simulink model "C1"  (Simulink 7.4)
settings: Solver=ode45  StartTime=0.0  StopTime=30  MaxStep=0.1  AbsTol=1e-14
settings Model: Creator=Administrator  LastModifiedBy=Administrator

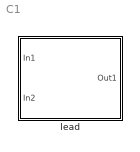
== system C1 ==
  lead : Subsystem

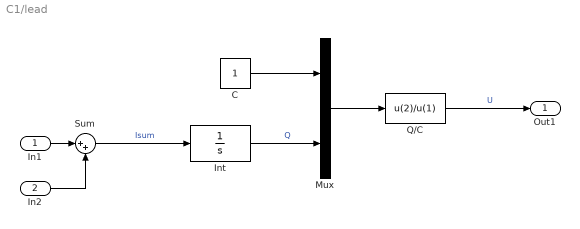
== system C1/lead ==
  In1 : Inport
  In2 : Inport  Port=2
  C : Constant  OutDataType=fixdt(1, 16)  OutScaling=2^0
  Int : Integrator
  Mux : Mux  Inputs=2
  Q/C : Fcn  Expr=u(2)/u(1)
  Sum : Sum  Inputs=|++  OutDataType=fixdt(1, 16)  OutScaling=2^0
  Out1 : Outport
  wires:
  Sum/1 -> Int/1  "Isum"
  Mux/1 -> Q/C/1
  C/1 -> Mux/1
  Int/1 -> Mux/2  "Q"
  Q/C/1 -> Out1/1  "U"
  In1/1 -> Sum/1
  In2/1 -> Sum/2
